simulink model "part3_datalog4_oldsimulink"  (R2018a)
settings: Solver=FixedStepAuto  StartTime=0.0  StopTime=count  FixedStep=1  RelTol=1e-3
libraries: simulink x1
settings Model: Creator=pete404  LastModifiedBy=pete404
settings DebuggingCC: LibraryContextMissingDiagnostic=warning
settings SFSimCC: SimUseLocalCustomCode=on
settings RTWCC: RTWUseLocalCustomCode=on

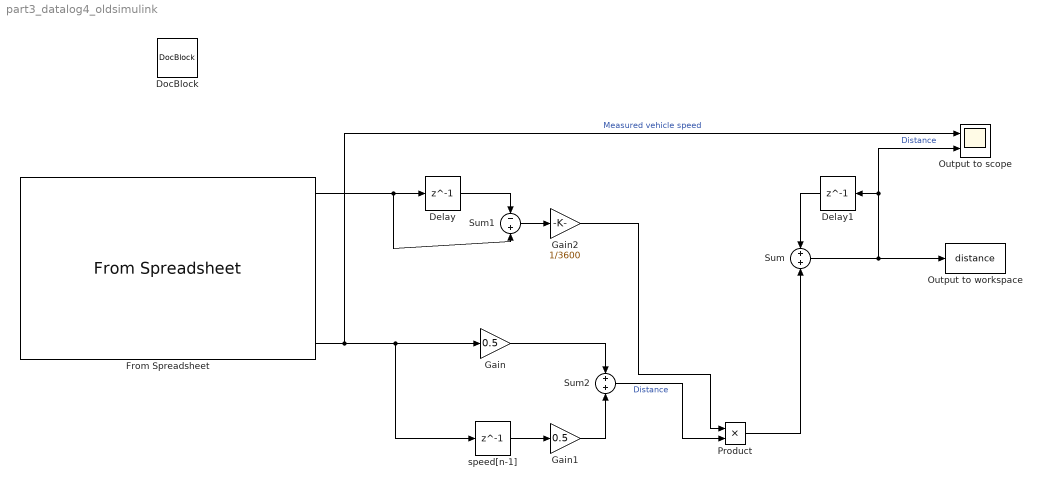
== system part3_datalog4_oldsimulink ==
  Delay : Delay  DelayLength=1  InitialCondition=0
  Delay1 : Delay  DelayLength=1  InitialCondition=0
  DocBlock : simulink/Model-Wide Utilities/DocBlock  DocumentType=Text
      content=|
      | Type your documentation here:
      |
      | Author: Peter A. Dranishnikov
      | Lab #: 5
      | Course: EEL 4685C
      | Due date: March 19th, Spring 2019
  From Spreadsheet : FromSpreadsheet  FileName=datalog4.xlsx  SheetName=datalog4
  Gain : Gain  Gain=0.5
  Gain1 : Gain  Gain=0.5
  Gain2 : Gain  Gain=1/3600
  Output to scope : Scope  NumInputPorts=2
  Output to workspace : ToWorkspace  VariableName=distance  SampleTime=-1
      settings: Save2DSignal=2-D array (concatenate along first dimension)
  Product : Product  OutDataTypeStr=double  RndMeth=Nearest
  Sum : Sum  AccumDataTypeStr=double  OutDataTypeStr=double  RndMeth=Nearest
  Sum1 : Sum  Inputs=-+  AccumDataTypeStr=double  OutDataTypeStr=double  RndMeth=Nearest
  Sum2 : Sum  AccumDataTypeStr=double  OutDataTypeStr=double  RndMeth=Nearest
  speed[n-1] : Delay  DelayLength=1  InitialCondition=0
  wires:
  From Spreadsheet/7 -> Output to scope/1, Gain/1, speed[n-1]/1  "Measured vehicle speed"
  Product/1 -> Sum/2
  From Spreadsheet/1 -> Delay/1, Sum1/2
  Delay/1 -> Sum1/1
  Sum/1 -> Delay1/1, Output to scope/2, Output to workspace/1  "Distance"
  Sum1/1 -> Gain2/1
  speed[n-1]/1 -> Gain1/1
  Gain2/1 -> Product/1
  Gain/1 -> Sum2/1
  Gain1/1 -> Sum2/2
  Sum2/1 -> Product/2  "Distance"
  Delay1/1 -> Sum/1
